simulink model "rSFCL_GitHub_Sim"  (R2019a)
settings: Solver=VariableStepAuto  StartTime=0.0  StopTime=0.1  MaxStep=1e-5  RelTol=1e-6
values from neighbouring files (symbols this model uses):
  Coefficient_temperature = 0.47e-8    (= 4.7e-09)    [rSFCL_GitHub.m]
  Cond_thermique_YBCO = 8    [rSFCL_GitHub.m]
  Critere_champ_Elec = 100e-6    (= 0.0001)    [rSFCL_GitHub.m]
  Ep_module_Ag_Bas = Ep_Ag_Bas / Nbr_module_Ep_Ag_Bas    (= 1.8e-06)    [rSFCL_GitHub.m]
  Ep_module_Ag_Haut = Ep_Ag_Haut / Nbr_module_Ep_Ag_Haut    (= 2e-06)    [rSFCL_GitHub.m]
  Ep_module_Hast = Ep_Hast / Nbr_module_Ep_Hast    (= 0.0001)    [rSFCL_GitHub.m]
  Ep_module_YBCO = Ep_YBCO / Nbr_module_Ep_YBCO    (= 1e-06)    [rSFCL_GitHub.m]
  Jc_critique = 2.5e10    (= 25000000000)    [rSFCL_GitHub.m]
  Largeur_ruban = 4e-3    (= 0.004)    [rSFCL_GitHub.m]
  Longeur_module = Longueur_ruban_sain / Nombre_module_sain    (= 10)    [rSFCL_GitHub.m]
  MV_argent = 10490    [rSFCL_GitHub.m]
  MV_hast = 8890    [rSFCL_GitHub.m]
  MV_YBCO = 6410    [rSFCL_GitHub.m]
  n_supra = 15    [rSFCL_GitHub.m]
  Res_inter_sain = Rho_interface * Epaisseur_R_int / Surface_sain    (= 2.5e-10)    [rSFCL_GitHub.m]
  Resisitance_etat_normal = 30e-8    (= 3e-07)    [rSFCL_GitHub.m]
  Temp_azote_liquide = 77    [rSFCL_GitHub.m]
  Temp_critique_supra = 90    [rSFCL_GitHub.m]
libraries: fl_lib x146, nesl_utility x87, ee_lib x5
(part 2 of 2)

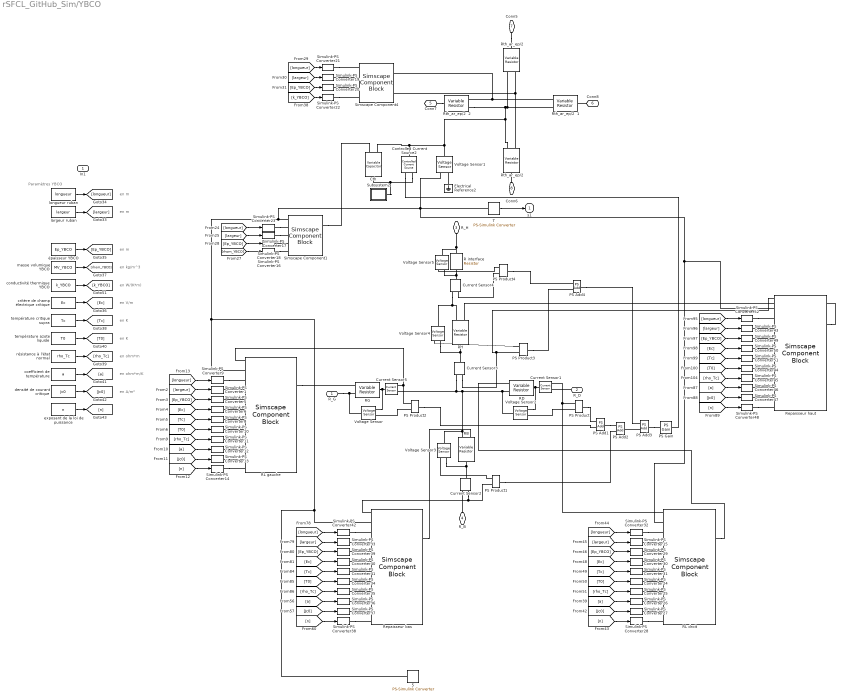
== system rSFCL_GitHub_Sim/YBCO  ==
  note: en ohm*m
  note: en m
  note: en kg/m^3
  note: en K
  note: Paramètres YBCO
  note: en K
  note: en V/m
  note: en W/(K*m)
  note: en m
  note: en m
  note: en ohm*m/K
  note: en A/m²
  In1 : Inport
  "    5" : nesl_utility/PS-Simulink Converter  PhysicalDomain=network_engine_domain  SubClassName=ps_output  LeftPortType=input  RightPortType=output  PseudoPeriodic=off  Frequencies=[]  Unit=1  AffineConversion=off
  Controlled Current Source2 : fl_lib/Electrical/Electrical Sources/Controlled Current Source
  Cth : ee_lib/Passive/Variable Capacitor  prm=2  Cmin=1e-9 F  r=1e-6 Ohm  v0=0 V  q0=0 C
      settings: SourceProductName=Simscape Electrical  SourceProductBaseCode=PS
  Current Sensor{1..5} (5 alike) : fl_lib/Electrical/Electrical Sensors/Current Sensor
  Electrical Reference2 : fl_lib/Electrical/Electrical Elements/Electrical Reference
  PS Add{1..4} (4 alike) : fl_lib/Physical Signals/Functions/PS Add
  PS Gain : fl_lib/Physical Signals/Functions/PS Gain  gain=1 1/V
  PS Product{,1..4} (5 alike) : fl_lib/Physical Signals/Functions/PS Product
      settings: SourceProductName=Simscape
  R interface : ee_lib/Passive/Resistor  R=Res_inter_sain Ohm  R_tol=5  enable_R_tol=0  tol_distribution=1  nSigma=4  enable_operating_limits=0  operating_limit_action=2  max_working_voltage=100 V  power_rating=1 W  enable_faults=0  fault_action=1  R_faulted=inf Ohm  enable_temporal_fault=0  t_fault=1 s  enable_behavioral_fault=0  max_permissible_current=1 A  t_fail_on_current=1 s  noise_mode=0  sample_time=1e-3 s  repeatability=1  auto_seed=3691276595  user_seed=0  Tdevice=25 degC  alpha=3.93e-3 1/K  Tmeas=25 degC  thermal_mass=100 J/K  power_derating_T1=70 degC  power_derating_T2=155 degC  operating_temperature_range_vec=[-50, 150] degC  temperature_specify=off  temperature_priority=High  temperature=298.15 K  temperature_nominal_specify=off  temperature_nominal_unit=K  temperature_nominal_value=1
      settings: SourceProductName=Simscape Electrical
  RB : fl_lib/Electrical/Electrical Elements/Variable Resistor  Rmin=RY Ohm  i_specify=off  i_priority=None  i=500 A  i_nominal_specify=off  i_nominal_unit=A  i_nominal_value=1  v_specify=off  v_priority=None  v=0 V  v_nominal_specify=off  v_nominal_unit=V  v_nominal_value=1
  RD : fl_lib/Electrical/Electrical Elements/Variable Resistor  Rmin=RY Ohm  i_specify=off  i_priority=None  i=500 A  i_nominal_specify=off  i_nominal_unit=A  i_nominal_value=1  v_specify=off  v_priority=None  v=0 V  v_nominal_specify=off  v_nominal_unit=V  v_nominal_value=1
  RG : fl_lib/Electrical/Electrical Elements/Variable Resistor  Rmin=RY Ohm  i_specify=off  i_priority=None  i=500 A  i_nominal_specify=off  i_nominal_unit=A  i_nominal_value=1  v_specify=off  v_priority=None  v=0 V  v_nominal_specify=off  v_nominal_unit=V  v_nominal_value=1
  RH : fl_lib/Electrical/Electrical Elements/Variable Resistor  Rmin=RY Ohm  i_specify=off  i_priority=None  i=500 A  i_nominal_specify=off  i_nominal_unit=A  i_nominal_value=1  v_specify=off  v_priority=None  v=0 V  v_nominal_specify=off  v_nominal_unit=V  v_nominal_value=1
  RL droit : SimscapeComponentBlock  SourceFile=Res_Elec_YBCO_L  ComponentPath=Res_Elec_YBCO_L  ComponentVariants=Res_Elec_YBCO_L  ComponentVariantNames=Res_Elec_YBCO_L  ClassName=Res_Elec_YBCO_L  SchemaVersion=1
      settings: CopyFcn=simscape.engine.sli.internal.componentblockcallback(gcbh,'COPY')  PreCopyFcn=simscape.engine.sli.internal.componentblockcallback(gcbh,'PRECOPY')  PreDeleteFcn=simscape.engine.sli.internal.componentblockcallback(gcbh,'PREDELETE')
      mask Type: UseFunction1
  RL gauche : SimscapeComponentBlock  SourceFile=Res_Elec_YBCO_L  ComponentPath=Res_Elec_YBCO_L  ComponentVariants=Res_Elec_YBCO_L  ComponentVariantNames=Res_Elec_YBCO_L  ClassName=Res_Elec_YBCO_L  SchemaVersion=1
      settings: CopyFcn=simscape.engine.sli.internal.componentblockcallback(gcbh,'COPY')  PreCopyFcn=simscape.engine.sli.internal.componentblockcallback(gcbh,'PRECOPY')  PreDeleteFcn=simscape.engine.sli.internal.componentblockcallback(gcbh,'PREDELETE')
      mask Type: UseFunction1
  Repaisseur bas : SimscapeComponentBlock  SourceFile=Res_Elec_YBCO_Ep  ComponentPath=Res_Elec_YBCO_Ep  ComponentVariants=Res_Elec_YBCO_Ep  ComponentVariantNames=Res_Elec_YBCO_Ep  ClassName=Res_Elec_YBCO_Ep  SchemaVersion=1
      settings: CopyFcn=simscape.engine.sli.internal.componentblockcallback(gcbh,'COPY')  PreCopyFcn=simscape.engine.sli.internal.componentblockcallback(gcbh,'PRECOPY')  PreDeleteFcn=simscape.engine.sli.internal.componentblockcallback(gcbh,'PREDELETE')
      mask Type: UseFunction1
  Repaisseur haut : SimscapeComponentBlock  SourceFile=Res_Elec_YBCO_Ep  ComponentPath=Res_Elec_YBCO_Ep  ComponentVariants=Res_Elec_YBCO_Ep  ComponentVariantNames=Res_Elec_YBCO_Ep  ClassName=Res_Elec_YBCO_Ep  SchemaVersion=1
      settings: CopyFcn=simscape.engine.sli.internal.componentblockcallback(gcbh,'COPY')  PreCopyFcn=simscape.engine.sli.internal.componentblockcallback(gcbh,'PRECOPY')  PreDeleteFcn=simscape.engine.sli.internal.componentblockcallback(gcbh,'PREDELETE')
      mask Type: UseFunction1
  "Rth_ar_ep/2  " : fl_lib/Electrical/Electrical Elements/Variable Resistor  Rmin=RY Ohm  i_specify=off  i_priority=None  i=500 A  i_nominal_specify=off  i_nominal_unit=A  i_nominal_value=1  v_specify=off  v_priority=None  v=0 V  v_nominal_specify=off  v_nominal_unit=V  v_nominal_value=1
  "Rth_ar_ep/2    " : fl_lib/Electrical/Electrical Elements/Variable Resistor  Rmin=RY Ohm  i_specify=off  i_priority=None  i=500 A  i_nominal_specify=off  i_nominal_unit=A  i_nominal_value=1  v_specify=off  v_priority=None  v=0 V  v_nominal_specify=off  v_nominal_unit=V  v_nominal_value=1
  Rth_ar_ep/2  1 : fl_lib/Electrical/Electrical Elements/Variable Resistor  Rmin=RY Ohm  i_specify=off  i_priority=None  i=500 A  i_nominal_specify=off  i_nominal_unit=A  i_nominal_value=1  v_specify=off  v_priority=None  v=0 V  v_nominal_specify=off  v_nominal_unit=V  v_nominal_value=1
  Rth_ar_ep/2  2 : fl_lib/Electrical/Electrical Elements/Variable Resistor  Rmin=RY Ohm  i_specify=off  i_priority=None  i=500 A  i_nominal_specify=off  i_nominal_unit=A  i_nominal_value=1  v_specify=off  v_priority=None  v=0 V  v_nominal_specify=off  v_nominal_unit=V  v_nominal_value=1
  Simscape Component1 : SimscapeComponentBlock  SourceFile=Cth_YBCO  ComponentPath=Cth_YBCO  ComponentVariants=Cth_YBCO  ComponentVariantNames=Cth_YBCO  ClassName=Cth_YBCO  SchemaVersion=1
      settings: CopyFcn=simscape.engine.sli.internal.componentblockcallback(gcbh,'COPY')  PreCopyFcn=simscape.engine.sli.internal.componentblockcallback(gcbh,'PRECOPY')  PreDeleteFcn=simscape.engine.sli.internal.componentblockcallback(gcbh,'PREDELETE')
      mask Type: UseFunction1
  Simscape Component4 : SimscapeComponentBlock  SourceFile=Rth_YBCO  ComponentPath=Rth_YBCO  ComponentVariants=Rth_YBCO  ComponentVariantNames=Rth_YBCO  ClassName=Rth_YBCO  SchemaVersion=1
      settings: CopyFcn=simscape.engine.sli.internal.componentblockcallback(gcbh,'COPY')  PreCopyFcn=simscape.engine.sli.internal.componentblockcallback(gcbh,'PRECOPY')  PreDeleteFcn=simscape.engine.sli.internal.componentblockcallback(gcbh,'PREDELETE')
      mask Type: UseFunction1
  Simulink-PS Converter{1,5..6,8..52} (48 alike) : nesl_utility/Simulink-PS Converter  PhysicalDomain=network_engine_domain  SubClassName=ps_input  LeftPortType=input  RightPortType=output  PseudoPeriodic=off  Frequencies=[]  NoiseDistribution=none  NoiseParameters=[]  Unit=1  AffineConversion=off  FilteringAndDerivatives=provide  SimscapeFilterOrder=1  InputFilterTimeConstant=0.001  UdotUserProvided=0
  Subsystem2 : Subsystem
  T : nesl_utility/PS-Simulink Converter  PhysicalDomain=network_engine_domain  SubClassName=ps_output  LeftPortType=input  RightPortType=output  PseudoPeriodic=off  Frequencies=[]  Unit=V  AffineConversion=off
  Voltage Sensor{,1..5} (6 alike) : fl_lib/Electrical/Electrical Sensors/Voltage Sensor
  coefficient de température : Constant  Value=a
  conductivité thermique YBCO : Constant  Value=k_YBCO
  critère de champ électrique critique : Constant  Value=Ec
  densité de courant critique : Constant  Value=Jc0
  exposant de la loi de puissance : Constant  Value=n
  largeur ruban : Constant  Value=largeur
  longueur ruban : Constant  Value=longueur
  masse volumique YBCO : Constant  Value=MV_YBCO
  résistance à l'état normal : Constant  Value=rho_Tc
  température azote liquide : Constant  Value=T0
  température critique supra : Constant  Value=Tc
  épaisseur YBCO : Constant  Value=Ep_YBCO
  R_G : PMIOPort  Side=Left
  R_D : PMIOPort  Port=2  Side=Right
  R_H : PMIOPort  Port=3  Side=Left
  R_B : PMIOPort  Port=4  Side=Right
  Conn7 : PMIOPort  Port=5  Side=Left
  Conn8 : PMIOPort  Port=6  Side=Right
  Conn5 : PMIOPort  Port=7  Side=Left
  Conn6 : PMIOPort  Port=8  Side=Right
  s1 : Outport
  wires:
  résistance à l'état normal/1 -> [rho_Tc]
  critère de champ électrique critique/1 -> [Ec]
  longueur ruban/1 -> [longueur]
  épaisseur YBCO/1 -> [Ep_YBCO]
  conductivité thermique YBCO/1 -> [k_YBCO]
  température critique supra/1 -> [Tc]
  température azote liquide/1 -> [T0]
  densité de courant critique/1 -> [Jc0]
  masse volumique YBCO/1 -> [rhom_YBCO]
  coefficient de température/1 -> [a]
  exposant de la loi de puissance/1 -> [n]
  largeur ruban/1 -> [largeur]
  [n] -> Simulink-PS Converter14/1
  [Jc0] -> Simulink-PS Converter13/1
  [a] -> Simulink-PS Converter12/1
  [rho_Tc] -> Simulink-PS Converter11/1
  [T0] -> Simulink-PS Converter10/1
  [Tc] -> Simulink-PS Converter8/1
  [Ec] -> Simulink-PS Converter6/1
  [Ep_YBCO] -> Simulink-PS Converter5/1
  [largeur] -> Simulink-PS Converter1/1
  [longueur] -> Simulink-PS Converter9/1
  [rhom_YBCO] -> Simulink-PS Converter16/1
  [largeur] -> Simulink-PS Converter17/1
  [Ep_YBCO] -> Simulink-PS Converter18/1
  [Ep_YBCO] -> Simulink-PS Converter20/1
  [longueur] -> Simulink-PS Converter23/1
  [largeur] -> Simulink-PS Converter19/1
  [longueur] -> Simulink-PS Converter21/1
  [k_YBCO] -> Simulink-PS Converter22/1
  [a] -> Simulink-PS Converter26/1
  [n] -> Simulink-PS Converter28/1
  [Tc] -> Simulink-PS Converter31/1
  [longueur] -> Simulink-PS Converter32/1
  [largeur] -> Simulink-PS Converter15/1
  [Jc0] -> Simulink-PS Converter27/1
  [Ep_YBCO] -> Simulink-PS Converter29/1
  [T0] -> Simulink-PS Converter24/1
  [rho_Tc] -> Simulink-PS Converter25/1
  [Ec] -> Simulink-PS Converter30/1
  [Ec] -> Simulink-PS Converter40/1
  [Tc] -> Simulink-PS Converter41/1
  [longueur] -> Simulink-PS Converter42/1
  [a] -> Simulink-PS Converter36/1
  [Ep_YBCO] -> Simulink-PS Converter39/1
  [largeur] -> Simulink-PS Converter33/1
  [Jc0] -> Simulink-PS Converter37/1
  [T0] -> Simulink-PS Converter34/1
  [rho_Tc] -> Simulink-PS Converter35/1
  [n] -> Simulink-PS Converter38/1
  [n] -> Simulink-PS Converter48/1
  [T0] -> Simulink-PS Converter44/1
  [Jc0] -> Simulink-PS Converter47/1
  [largeur] -> Simulink-PS Converter43/1
  [rho_Tc] -> Simulink-PS Converter45/1
  [Ep_YBCO] -> Simulink-PS Converter49/1
  [longueur] -> Simulink-PS Converter52/1
  [a] -> Simulink-PS Converter46/1
  [Ec] -> Simulink-PS Converter50/1
  [Tc] -> Simulink-PS Converter51/1
  T/1 -> s1/1
  connections:
  Simulink-PS Converter9/RConn1 -- RL gauche/LConn3
  Simulink-PS Converter1/RConn1 -- RL gauche/LConn4
  Simulink-PS Converter5/RConn1 -- RL gauche/LConn5
  Simulink-PS Converter6/RConn1 -- RL gauche/LConn6
  Simulink-PS Converter8/RConn1 -- RL gauche/LConn7
  Simulink-PS Converter10/RConn1 -- RL gauche/LConn8
  Simulink-PS Converter11/RConn1 -- RL gauche/LConn9
  Simulink-PS Converter12/RConn1 -- RL gauche/LConn10
  Simulink-PS Converter13/RConn1 -- RL gauche/LConn11
  Simulink-PS Converter14/RConn1 -- RL gauche/LConn12
  Simulink-PS Converter20/RConn1 -- Simscape Component4/LConn3
  Simulink-PS Converter23/RConn1 -- Simscape Component1/LConn2
  Simulink-PS Converter16/RConn1 -- Simscape Component1/LConn5
  Simulink-PS Converter17/RConn1 -- Simscape Component1/LConn3
  Simulink-PS Converter18/RConn1 -- Simscape Component1/LConn4
  Simulink-PS Converter22/RConn1 -- Simscape Component4/LConn4
  Simulink-PS Converter19/RConn1 -- Simscape Component4/LConn2
  Simulink-PS Converter21/RConn1 -- Simscape Component4/LConn1
  Simulink-PS Converter31/RConn1 -- RL droit/LConn7
  Simulink-PS Converter26/RConn1 -- RL droit/LConn10
  Simulink-PS Converter25/RConn1 -- RL droit/LConn9
  Simulink-PS Converter27/RConn1 -- RL droit/LConn11
  Simulink-PS Converter15/RConn1 -- RL droit/LConn4
  Simulink-PS Converter24/RConn1 -- RL droit/LConn8
  Simulink-PS Converter29/RConn1 -- RL droit/LConn5
  Simulink-PS Converter28/RConn1 -- RL droit/LConn12
  Simulink-PS Converter30/RConn1 -- RL droit/LConn6
  Simulink-PS Converter32/RConn1 -- RL droit/LConn3
  Simulink-PS Converter41/RConn1 -- Repaisseur bas/LConn7
  Simulink-PS Converter42/RConn1 -- Repaisseur bas/LConn3
  Simulink-PS Converter36/RConn1 -- Repaisseur bas/LConn10
  Simulink-PS Converter33/RConn1 -- Repaisseur bas/LConn4
  Simulink-PS Converter38/RConn1 -- Repaisseur bas/LConn12
  Simulink-PS Converter34/RConn1 -- Repaisseur bas/LConn8
  Simulink-PS Converter40/RConn1 -- Repaisseur bas/LConn6
  Simulink-PS Converter37/RConn1 -- Repaisseur bas/LConn11
  Simulink-PS Converter35/RConn1 -- Repaisseur bas/LConn9
  Simulink-PS Converter39/RConn1 -- Repaisseur bas/LConn5
  Simulink-PS Converter48/RConn1 -- Repaisseur haut/LConn12
  Simulink-PS Converter45/RConn1 -- Repaisseur haut/LConn9
  Simulink-PS Converter49/RConn1 -- Repaisseur haut/LConn5
  Simulink-PS Converter43/RConn1 -- Repaisseur haut/LConn4
  Simulink-PS Converter47/RConn1 -- Repaisseur haut/LConn11
  Simulink-PS Converter50/RConn1 -- Repaisseur haut/LConn6
  Simulink-PS Converter44/RConn1 -- Repaisseur haut/LConn8
  Simulink-PS Converter52/RConn1 -- Repaisseur haut/LConn3
  Simulink-PS Converter46/RConn1 -- Repaisseur haut/LConn10
  Simulink-PS Converter51/RConn1 -- Repaisseur haut/LConn7
  R_B/RConn1 -- Current Sensor2/RConn2
  Cth/RConn1 -- Controlled Current Source2/RConn2 -- Subsystem2/LConn1
  Rth_ar_ep/2  1/LConn1 -- Rth_ar_ep/2  2/LConn1 -- Simscape Component4/RConn1
  Current Sensor5/LConn1 -- Voltage Sensor/RConn2 -- RG/RConn1
  Current Sensor1/LConn1 -- Voltage Sensor2/RConn2 -- RD/RConn1
  Voltage Sensor/LConn1 -- RG/LConn2 -- R_G/RConn1
  Voltage Sensor1/RConn1 -- T/LConn1 -- Repaisseur haut/LConn2 -- RL droit/LConn2 -- Simscape Component1/LConn1 -- RL gauche/LConn2 -- Repaisseur bas/LConn2 -- "    5"/LConn1
  Simscape Component1/RConn1 -- Cth/LConn1
  "Rth_ar_ep/2    "/LConn1 -- "Rth_ar_ep/2  "/LConn1 -- Simscape Component4/RConn2
  PS Add3/LConn2 -- PS Add2/RConn1
  Current Sensor3/RConn1 -- Repaisseur haut/LConn1 -- PS Product3/LConn2
  PS Product3/LConn1 -- Voltage Sensor4/RConn1
  PS Product1/RConn1 -- PS Add2/LConn2
  PS Add1/RConn1 -- PS Add2/LConn1
  Controlled Current Source2/RConn1 -- PS Gain/RConn1
  Conn7/RConn1 -- Rth_ar_ep/2  2/RConn1
  R_D/RConn1 -- Current Sensor1/RConn2
  RL droit/LConn1 -- PS Product/LConn1 -- Current Sensor1/RConn1
  Electrical Reference2/LConn1 -- Voltage Sensor1/RConn2
  Repaisseur bas/LConn1 -- Current Sensor2/RConn1 -- PS Product1/LConn2
  PS Product2/LConn2 -- Voltage Sensor/RConn1
  PS Product1/LConn1 -- Voltage Sensor3/RConn1
  PS Product2/LConn1 -- Current Sensor5/RConn1 -- RL gauche/LConn1
  PS Product/RConn1 -- PS Add1/LConn1
  PS Product/LConn2 -- Voltage Sensor2/RConn1
  PS Product2/RConn1 -- PS Add1/LConn2
  PS Add3/RConn1 -- PS Gain/LConn1
  Conn8/RConn1 -- Rth_ar_ep/2  1/RConn1
  RL gauche/RConn1 -- RG/LConn1
  RL droit/RConn1 -- RD/LConn1
  Repaisseur haut/RConn1 -- RH/LConn1
  Repaisseur bas/RConn1 -- RB/LConn1
  Current Sensor3/LConn1 -- Voltage Sensor4/RConn2 -- RH/RConn1
  Voltage Sensor3/RConn2 -- Current Sensor2/LConn1 -- RB/RConn1
  RH/LConn2 -- Current Sensor4/RConn2 -- Voltage Sensor4/LConn1
  RD/LConn2 -- Voltage Sensor3/LConn1 -- RB/LConn2 -- Current Sensor3/RConn2 -- Current Sensor5/RConn2 -- Voltage Sensor2/LConn1
  Conn6/RConn1 -- "Rth_ar_ep/2    "/RConn1
  R interface/LConn1 -- Voltage Sensor5/LConn1 -- R_H/RConn1
  Current Sensor4/LConn1 -- Voltage Sensor5/RConn2 -- R interface/RConn1
  Current Sensor4/RConn1 -- PS Product4/LConn2
  PS Product4/LConn1 -- Voltage Sensor5/RConn1
  PS Product4/RConn1 -- PS Add4/LConn1
  PS Product3/RConn1 -- PS Add4/LConn2
  PS Add4/RConn1 -- PS Add3/LConn1
  Controlled Current Source2/LConn1 -- Rth_ar_ep/2  1/LConn2 -- "Rth_ar_ep/2  "/LConn2 -- Rth_ar_ep/2  2/LConn2 -- "Rth_ar_ep/2    "/LConn2 -- Voltage Sensor1/LConn1 -- Cth/LConn2
  Conn5/RConn1 -- "Rth_ar_ep/2  "/RConn1

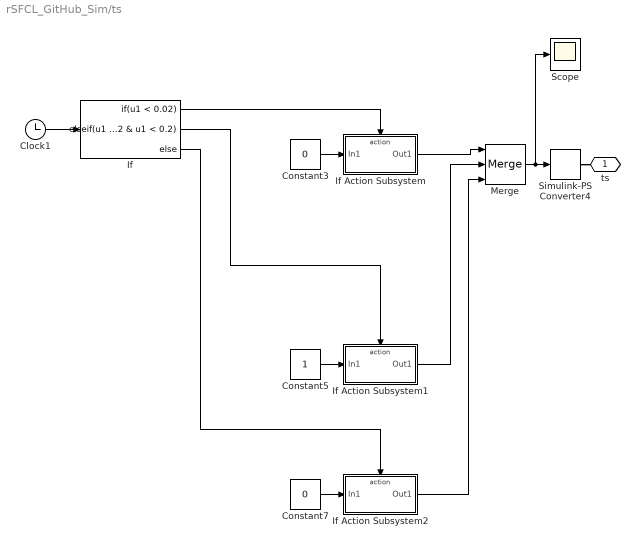
== system rSFCL_GitHub_Sim/ts ==
  Clock1 : Clock
  Constant3 : Constant  Value=0
  Constant5 : Constant
  Constant7 : Constant  Value=0
  If : If  IfExpression=u1 < 0.02  ElseIfExpressions=u1 >= 0.02 & u1 < 0.2
  If Action Subsystem : Subsystem  TreatAsAtomicUnit=on
  If Action Subsystem1 : Subsystem  TreatAsAtomicUnit=on
  If Action Subsystem2 : Subsystem  TreatAsAtomicUnit=on
  Merge : Merge  Inputs=3
  Scope : Scope
  Simulink-PS Converter4 : nesl_utility/Simulink-PS Converter  PhysicalDomain=network_engine_domain  SubClassName=ps_input  LeftPortType=input  RightPortType=output  PseudoPeriodic=off  Frequencies=[]  NoiseDistribution=none  NoiseParameters=[]  Unit=1  AffineConversion=off  FilteringAndDerivatives=provide  SimscapeFilterOrder=1  InputFilterTimeConstant=0.001  UdotUserProvided=0
  ts : PMIOPort  Side=Right
  wires:
  Merge/1 -> Scope/1, Simulink-PS Converter4/1
  Constant3/1 -> If Action Subsystem/1(In1)
  If Action Subsystem/1(Out1) -> Merge/1
  If Action Subsystem1/1(Out1) -> Merge/2
  Constant5/1 -> If Action Subsystem1/1(In1)
  Constant7/1 -> If Action Subsystem2/1(In1)
  If Action Subsystem2/1(Out1) -> Merge/3
  Clock1/1 -> If/1
  If/1 -> If Action Subsystem/Action
  If/2 -> If Action Subsystem1/Action
  If/3 -> If Action Subsystem2/Action
  connections:
  Simulink-PS Converter4/RConn1 -- ts/RConn1

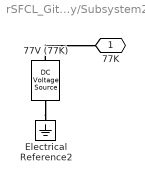
== system rSFCL_GitHub_Sim/Hastelloy/Subsystem2 ==
  77V (77K) : fl_lib/Electrical/Electrical Sources/DC Voltage Source  v0=77 V
  Electrical Reference2 : fl_lib/Electrical/Electrical Elements/Electrical Reference
  "77K " : PMIOPort  Side=Left
  connections:
  77V (77K)/LConn1 -- "77K "/RConn1
  77V (77K)/RConn1 -- Electrical Reference2/LConn1

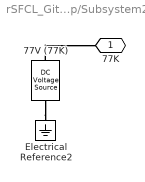
== system rSFCL_GitHub_Sim/Silver Top/Subsystem2 ==
  77V (77K) : fl_lib/Electrical/Electrical Sources/DC Voltage Source  v0=77 V
  Electrical Reference2 : fl_lib/Electrical/Electrical Elements/Electrical Reference
  "77K " : PMIOPort  Side=Left
  connections:
  77V (77K)/LConn1 -- "77K "/RConn1
  77V (77K)/RConn1 -- Electrical Reference2/LConn1

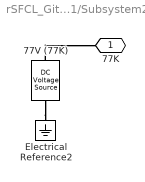
== system rSFCL_GitHub_Sim/Silver Top1/Subsystem2 ==
  77V (77K) : fl_lib/Electrical/Electrical Sources/DC Voltage Source  v0=77 V
  Electrical Reference2 : fl_lib/Electrical/Electrical Elements/Electrical Reference
  "77K " : PMIOPort  Side=Left
  connections:
  77V (77K)/LConn1 -- "77K "/RConn1
  77V (77K)/RConn1 -- Electrical Reference2/LConn1

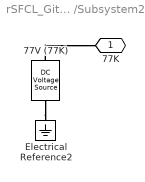
== system rSFCL_GitHub_Sim/YBCO /Subsystem2 ==
  77V (77K) : fl_lib/Electrical/Electrical Sources/DC Voltage Source  v0=77 V
  Electrical Reference2 : fl_lib/Electrical/Electrical Elements/Electrical Reference
  "77K " : PMIOPort  Side=Left
  connections:
  77V (77K)/LConn1 -- "77K "/RConn1
  77V (77K)/RConn1 -- Electrical Reference2/LConn1

== system rSFCL_GitHub_Sim/ts/If Action Subsystem ==
  In1 : Inport
  Action Port : ActionPort  ActionPortLabel=if(u1 < 0.02)
  Out1 : Outport
  wires:
  In1/1 -> Out1/1

== system rSFCL_GitHub_Sim/ts/If Action Subsystem1 ==
  In1 : Inport
  Action Port : ActionPort  ActionPortLabel=elseif(u1 >= 0.02 & u1 < 0.2)
  Out1 : Outport
  wires:
  In1/1 -> Out1/1

== system rSFCL_GitHub_Sim/ts/If Action Subsystem2 ==
  In1 : Inport
  Action Port : ActionPort  ActionPortLabel=else
  Out1 : Outport
  wires:
  In1/1 -> Out1/1
